simulink model "six_dof_dynamics"  (R2024b)
settings: Solver=VariableStepAuto  StartTime=0.0  StopTime=10.0  RelTol=1e-3
undefined symbols (not defined in the file or in its folder): armTVC, c_d, contact, g, m, tf_tvc
libraries: simulink_extras x2, shared6dof x1, simulink x1, sharedtransform x1, sharedutil x1, uavutilslib x1
settings Model: Creator=tommy  LastModifiedBy=tommy

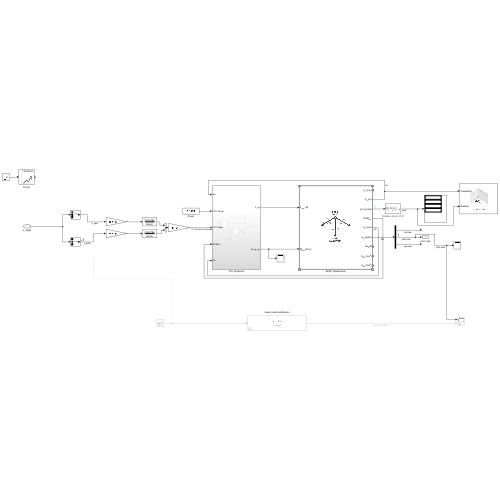
[thumbnail: Simulink's stored preview of the top-level diagram]
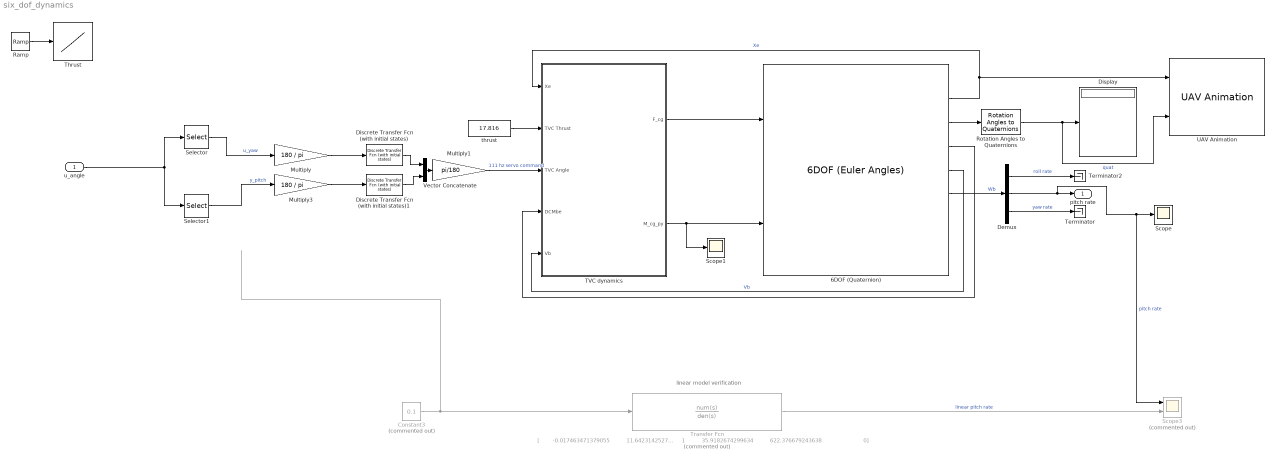
== system six_dof_dynamics ==
  note: linear model verification
  u_angle : Inport
  6DOF (Quaternion) : shared6dof/6DOF (Euler Angles)  units=Metric (MKS)  mtype=Fixed  rep=Quaternion  xme_0=[0 0 0]  Vm_0=[0 0 0]  eul_0=initial_euler  pm_0=[0 0 0]  mass_0=m  mass_e=0.5  mass_f=2.0  inertia=inertia  inertia_e=eye(3)  inertia_f=2*eye(3)  k_quat=1  vre_flag=on  abi_flag=on  aMode=0  xme_statename=''  Vm_statename=''  eul_statename=''  quat_statename=''  pm_statename=''  mass_statename=''
  Constant3 : Constant  Commented=on  Value=0.1
  Demux : Demux  Outputs=3
  Discrete Transfer Fcn (with initial states) : simulink_extras/Additional Discrete/Discrete Transfer Fcn (with initial states)  N=tf_tvc.Numerator  D=tf_tvc.Denominator  X0=0  TS=tf_tvc.Ts
  Discrete Transfer Fcn (with initial states)1 : simulink_extras/Additional Discrete/Discrete Transfer Fcn (with initial states)  N=tf_tvc.Numerator  D=tf_tvc.Denominator  X0=0  TS=tf_tvc.Ts
  Display : Display
  Multiply : Gain  Gain=180 / pi
  Multiply1 : Gain  Gain=pi/180
  Multiply3 : Gain  Gain=180 / pi
  Ramp : simulink/Sources/Ramp  slope=1  start=0  InitialOutput=0
  Rotation Angles to Quaternions : sharedtransform/Rotation Angles to Quaternions  rotationOrder=XYZ  aMode=aMode
  Scope : Scope
  Scope1 : Scope
  Scope3 : Scope  Commented=on  NumInputPorts=2
  Selector : Selector  InputPortWidth=3  IndexOptions=Index vector (dialog)  Indices=[1]  OutputSizes=1
  Selector1 : Selector  InputPortWidth=3  IndexOptions=Index vector (dialog)  Indices=[2]  OutputSizes=1
  TVC dynamics : Subsystem
  Terminator : Terminator
  Terminator2 : Terminator
  Thrust : Lookup_n-D  NumberOfTableDimensions=1  BreakpointsForDimension1=[0;0.15;0.186;0.206;0.242;0.252;0.277;0.333;0.359;0.374;0.394;0.435;0.476;0.521;0.643;0.725;0.821;0.898;1.025;1.142;1.259;1.396;1.569;1.757;1.895;2.027;2.042;2.052;2.063;2.09;4;10]  Table=[0;1.371;1.92;3.387;5.587;7.422;8.705;13.474;15.858;16.592;18.609;21.544;24.661;26.44;21.72;20.432;19.511;18.958;18.219;18.032;17.844;17.472;17.282;17.275;17.086;17.816;12.494;8.457;4.97;0;0;0]  InterpMethod=Akima spline  InternalRulePriority=Speed  RndMeth=Simplest
  Transfer Fcn : TransferFcn  Commented=on  Numerator="[        -0.017463471379055          11.6423142527021         -2587.18094504468          191643.032966257]"  Denominator="[                         1          35.9182674299634          622.376679243638                         0]"
  UAV Animation : uavutilslib/UAV Animation  NumUAV=1  DynamicUAVConfig=off  UAVType=FixedWing  UAVSize=1  UAVColor=[1 0 0]  UAVTrajectoryAlpha=1  InertialZDirection=Down  RotationFormat=Quaternion  DrawMarkers=off  SampleTime=-1
  Vector Concatenate : Concatenate
  thrust : Constant  Value=17.816
  pitch rate : Outport
  wires:
  Rotation Angles to Quaternions/1 -> UAV Animation/2, Display/1  "quat"
  thrust/1 -> TVC dynamics/2(TVC Thrust)
  TVC dynamics/1(F_cg) -> 6DOF (Quaternion)/1
  6DOF (Quaternion)/3 -> Rotation Angles to Quaternions/1
  TVC dynamics/2(M_cg_py) -> 6DOF (Quaternion)/2, Scope1/1
  6DOF (Quaternion)/2 -> UAV Animation/1, TVC dynamics/1(Xe)  "Xe"
  Discrete Transfer Fcn (with initial states)/1 -> Vector Concatenate/1
  6DOF (Quaternion)/5 -> TVC dynamics/5(Vb)  "Vb"
  6DOF (Quaternion)/4 -> TVC dynamics/4(DCMbe)
  Vector Concatenate/1 -> Multiply1/1
  6DOF (Quaternion)/6 -> Demux/1  "Wb"
  Multiply1/1 -> TVC dynamics/3(TVC Angle)  "111 hz servo command"
  Ramp/1 -> Thrust/1
  Demux/1 -> Terminator2/1  "roll rate"
  Demux/2 -> Scope3/1, Scope/1, pitch rate/1  "pitch rate"
  Demux/3 -> Terminator/1  "yaw rate"
  u_angle/1 -> Selector1/1, Selector/1
  Selector/1 -> Multiply/1  "u_yaw"
  Selector1/1 -> Multiply3/1  "y_pitch"
  Multiply/1 -> Discrete Transfer Fcn (with initial states)/1
  Transfer Fcn/1 -> Scope3/2  "linear pitch rate"
  Constant3/1 -> Transfer Fcn/1
  Multiply3/1 -> Discrete Transfer Fcn (with initial states)1/1
  Discrete Transfer Fcn (with initial states)1/1 -> Vector Concatenate/2

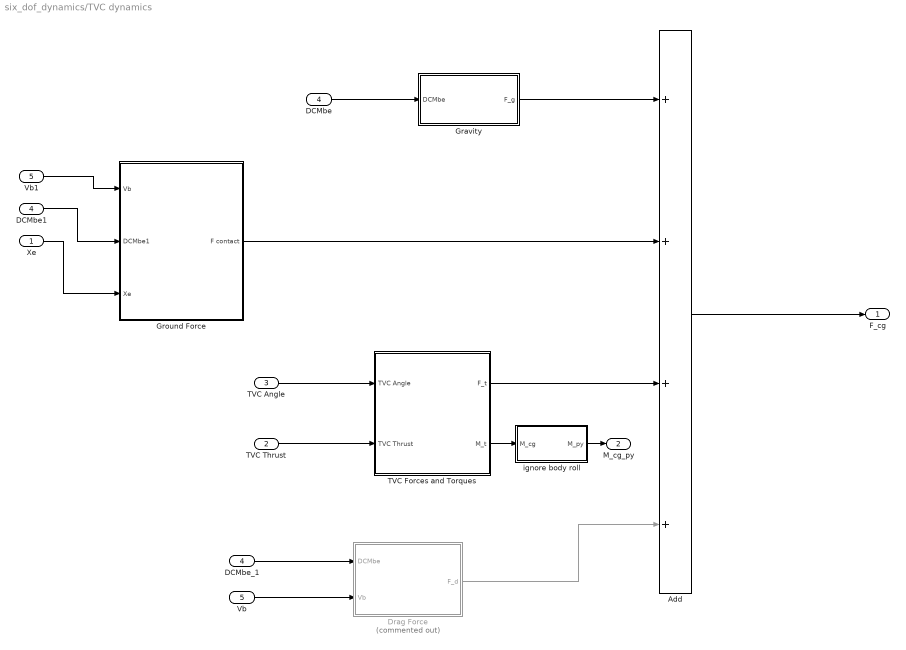
== system six_dof_dynamics/TVC dynamics ==
  Xe : Inport
  TVC Thrust : Inport  Port=2
  TVC Angle : Inport  Port=3
  DCMbe : Inport  Port=4
  Vb : Inport  Port=5
  Add : Sum  Inputs=++++
  DCMbe1 : InportShadow  Port=4
  DCMbe_1 : InportShadow  Port=4
  Drag Force : Subsystem  Commented=on
  Gravity : Subsystem
  Ground Force : Subsystem
  TVC Forces and Torques : Subsystem
  Vb1 : InportShadow  Port=5
  "ignore body roll " : Subsystem
  F_cg : Outport
  M_cg_py : Outport  Port=2
  wires:
  Add/1 -> F_cg/1
  DCMbe_1/1 -> Drag Force/1(DCMbe)
  TVC Forces and Torques/1(F_t) -> Add/3
  Vb/1 -> Drag Force/2(Vb)
  Gravity/1(F_g) -> Add/1
  TVC Thrust/1 -> TVC Forces and Torques/2(TVC Thrust)
  TVC Forces and Torques/2(M_t) -> "ignore body roll "/1(M_cg)
  DCMbe/1 -> Gravity/1(DCMbe)
  TVC Angle/1 -> TVC Forces and Torques/1(TVC Angle)
  Drag Force/1(F_d) -> Add/4
  DCMbe1/1 -> Ground Force/2(DCMbe1)
  Xe/1 -> Ground Force/3(Xe)
  Ground Force/1(F contact) -> Add/2
  Vb1/1 -> Ground Force/1(Vb)
  "ignore body roll "/1(M_py) -> M_cg_py/1

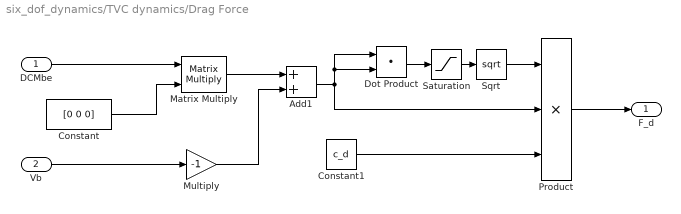
== system six_dof_dynamics/TVC dynamics/Drag Force ==
  DCMbe : Inport
  Vb : Inport  Port=2
  Add1 : Sum
  Constant : Constant  Value=[0 0 0]
  Constant1 : Constant  Value=c_d
  Dot Product : DotProduct  OutDataTypeStr=Inherit: Inherit via internal rule
  Matrix Multiply : Product  Multiplication=Matrix(*)
  Multiply : Gain  Gain=-1
  Product : Product  Inputs=3
  Saturation : Saturate  UpperLimit=inf  LowerLimit=0.00001
  Sqrt : Sqrt
  F_d : Outport
  wires:
  Dot Product/1 -> Saturation/1
  Multiply/1 -> Add1/2
  Constant/1 -> Matrix Multiply/2
  Matrix Multiply/1 -> Add1/1
  Add1/1 -> Product/2, Dot Product/1, Dot Product/2
  Vb/1 -> Multiply/1
  DCMbe/1 -> Matrix Multiply/1
  Sqrt/1 -> Product/1
  Saturation/1 -> Sqrt/1
  Product/1 -> F_d/1
  Constant1/1 -> Product/3

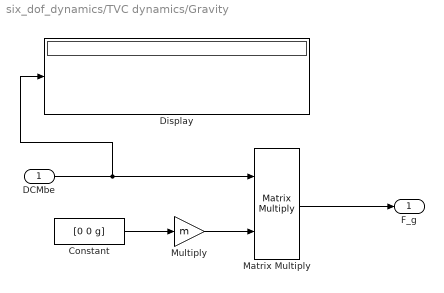
== system six_dof_dynamics/TVC dynamics/Gravity ==
  DCMbe : Inport
  Constant : Constant  Value=[0 0 g]
  Display : Display
  Matrix Multiply : Product  Multiplication=Matrix(*)
  Multiply : Gain  Gain=m
  F_g : Outport
  wires:
  Multiply/1 -> Matrix Multiply/2
  DCMbe/1 -> Display/1, Matrix Multiply/1
  Constant/1 -> Multiply/1
  Matrix Multiply/1 -> F_g/1

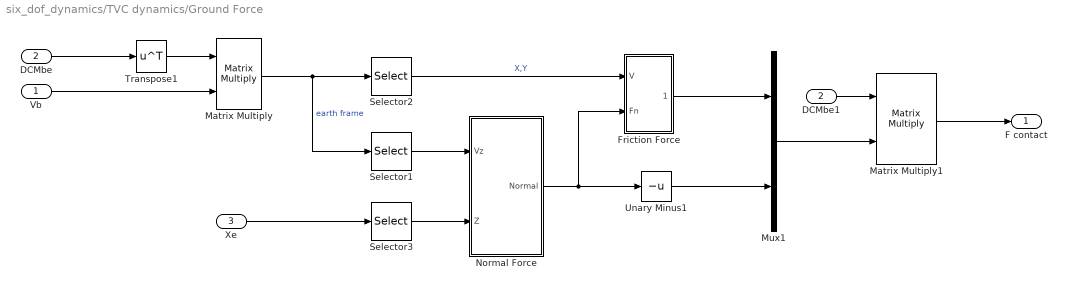
== system six_dof_dynamics/TVC dynamics/Ground Force ==
  Vb : Inport
  DCMbe1 : Inport  Port=2
  Xe : Inport  Port=3
  DCMbe : InportShadow  Port=2
  Friction Force : Subsystem
  Matrix Multiply : Product  Multiplication=Matrix(*)
  Matrix Multiply1 : Product  Multiplication=Matrix(*)
  Mux1 : Mux  Inputs=2
  Normal Force : Subsystem
  Selector1 : Selector  InputPortWidth=3  IndexOptions=Index vector (dialog)  Indices=[3]  OutputSizes=1
  Selector2 : Selector  InputPortWidth=3  IndexOptions=Index vector (dialog)  Indices=[1,2]  OutputSizes=1
  Selector3 : Selector  InputPortWidth=3  IndexOptions=Index vector (dialog)  Indices=[3]  OutputSizes=1
  Transpose1 : Math  Operator=transpose
  Unary Minus1 : UnaryMinus
  F contact : Outport
  wires:
  Matrix Multiply1/1 -> F contact/1
  Friction Force/1(Friction) -> Mux1/1
  Xe/1 -> Selector3/1
  Vb/1 -> Matrix Multiply/2
  Selector3/1 -> Normal Force/2(Z)
  Matrix Multiply/1 -> Selector1/1, Selector2/1  "earth frame"
  Mux1/1 -> Matrix Multiply1/2
  Selector2/1 -> Friction Force/1(V)  "X,Y"
  Selector1/1 -> Normal Force/1(Vz)
  DCMbe1/1 -> Matrix Multiply1/1
  DCMbe/1 -> Transpose1/1
  Transpose1/1 -> Matrix Multiply/1
  Unary Minus1/1 -> Mux1/2
  Normal Force/1(Normal) -> Unary Minus1/1, Friction Force/2(Fn)

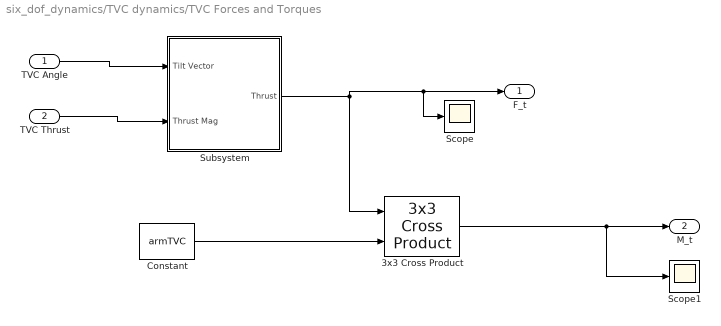
== system six_dof_dynamics/TVC dynamics/TVC Forces and Torques ==
  TVC Angle : Inport
  TVC Thrust : Inport  Port=2
  3x3 Cross Product : sharedutil/3x3 Cross Product  aMode=aMode
  Constant : Constant  Value=armTVC
  Scope : Scope
  Scope1 : Scope
  Subsystem : Subsystem
  F_t : Outport
  M_t : Outport  Port=2
  wires:
  TVC Angle/1 -> Subsystem/1(Tilt Vector)
  TVC Thrust/1 -> Subsystem/2(Thrust Mag)
  Subsystem/1(Thrust) -> Scope/1, F_t/1, 3x3 Cross Product/1
  Constant/1 -> 3x3 Cross Product/2
  3x3 Cross Product/1 -> Scope1/1, M_t/1

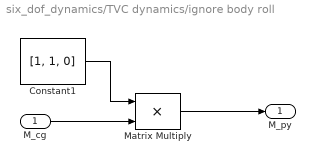
== system six_dof_dynamics/TVC dynamics/ignore body roll  ==
  M_cg : Inport
  Constant1 : Constant  Value=[1, 1, 0]
  Matrix Multiply : Product
  M_py : Outport
  wires:
  Constant1/1 -> Matrix Multiply/1
  Matrix Multiply/1 -> M_py/1
  M_cg/1 -> Matrix Multiply/2

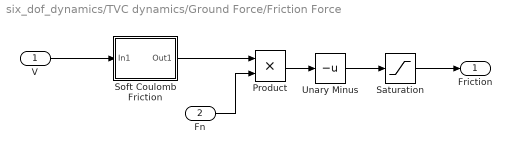
== system six_dof_dynamics/TVC dynamics/Ground Force/Friction Force ==
  V : Inport
  Fn : Inport  Port=2
  Product : Product
  Saturation : Saturate  UpperLimit=contact.translation.maxFriction  LowerLimit=-contact.translation.maxFriction
  Soft Coulomb Friction : Subsystem
  Unary Minus : UnaryMinus
  Friction : Outport
  wires:
  Fn/1 -> Product/2
  Soft Coulomb Friction/1(Out1) -> Product/1
  Product/1 -> Unary Minus/1
  V/1 -> Soft Coulomb Friction/1(In1)
  Unary Minus/1 -> Saturation/1
  Saturation/1 -> Friction/1

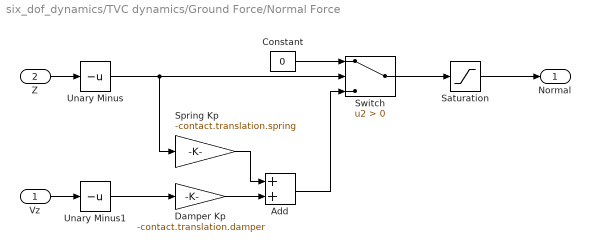
== system six_dof_dynamics/TVC dynamics/Ground Force/Normal Force ==
  Vz : Inport
  Z : Inport  Port=2
  Add : Sum
  Constant : Constant  Value=0
  Damper Kp : Gain  Gain=-contact.translation.damper
  Saturation : Saturate  UpperLimit=contact.translation.maxNormal  LowerLimit=0
  Spring Kp : Gain  Gain=-contact.translation.spring
  Switch : Switch  Criteria=u2 > Threshold  SaturateOnIntegerOverflow=off  InputSameDT=off
  Unary Minus : UnaryMinus
  Unary Minus1 : UnaryMinus
  Normal : Outport
  wires:
  Constant/1 -> Switch/1
  Z/1 -> Unary Minus/1
  Switch/1 -> Saturation/1
  Damper Kp/1 -> Add/2
  Add/1 -> Switch/3
  Spring Kp/1 -> Add/1
  Vz/1 -> Unary Minus1/1
  Saturation/1 -> Normal/1
  Unary Minus/1 -> Spring Kp/1, Switch/2
  Unary Minus1/1 -> Damper Kp/1

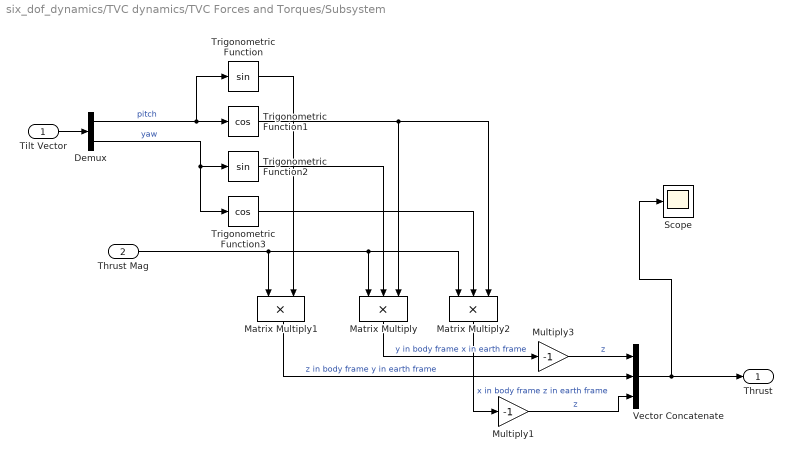
== system six_dof_dynamics/TVC dynamics/TVC Forces and Torques/Subsystem ==
  Tilt Vector : Inport
  Thrust Mag : Inport  Port=2
  Demux : Demux  Outputs=2
  Matrix Multiply : Product  Inputs=3
  Matrix Multiply1 : Product
  Matrix Multiply2 : Product  Inputs=3
  Multiply1 : Gain  Gain=-1
  Multiply3 : Gain  Gain=-1
  Scope : Scope
  Trigonometric Function : Trigonometry
  Trigonometric Function1 : Trigonometry  Operator=cos
  Trigonometric Function2 : Trigonometry
  Trigonometric Function3 : Trigonometry  Operator=cos
  Vector Concatenate : Concatenate  NumInputs=3
  Thrust : Outport
  wires:
  Demux/2 -> Trigonometric Function3/1, Trigonometric Function2/1  "yaw"
  Matrix Multiply1/1 -> Vector Concatenate/2  "z in body frame y in earth frame"
  Tilt Vector/1 -> Demux/1
  Trigonometric Function1/1 -> Matrix Multiply/3, Matrix Multiply2/3
  Demux/1 -> Trigonometric Function/1, Trigonometric Function1/1  "pitch"
  Trigonometric Function3/1 -> Matrix Multiply2/2
  Thrust Mag/1 -> Matrix Multiply2/1, Matrix Multiply/1, Matrix Multiply1/1
  Vector Concatenate/1 -> Scope/1, Thrust/1
  Matrix Multiply2/1 -> Multiply1/1  "x in body frame z in earth frame"
  Multiply1/1 -> Vector Concatenate/3  "z"
  Multiply3/1 -> Vector Concatenate/1  "z"
  Matrix Multiply/1 -> Multiply3/1  "y in body frame x in earth frame"
  Trigonometric Function/1 -> Matrix Multiply1/2
  Trigonometric Function2/1 -> Matrix Multiply/2

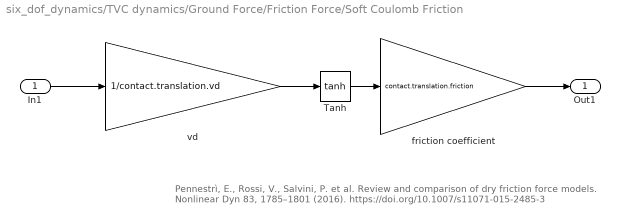
== system six_dof_dynamics/TVC dynamics/Ground Force/Friction Force/Soft Coulomb Friction ==
  note: Pennestrì, E., Rossi, V., Salvini, P. et al. Review and comparison of dry friction force models. Nonlinear Dyn 83, 1785–1801 (2016). https://doi.org/10.1007/s11071-015-2485-3
  In1 : Inport
  Tanh : Trigonometry  Operator=tanh
  friction coefficient : Gain  Gain=contact.translation.friction
  vd : Gain  Gain=1/contact.translation.vd
  Out1 : Outport
  wires:
  In1/1 -> vd/1
  vd/1 -> Tanh/1
  Tanh/1 -> friction coefficient/1
  friction coefficient/1 -> Out1/1
